simulink model "xo_test"  (R2023a)
settings: Solver=VariableStepAuto  StartTime=0.0  StopTime=10.0  RelTol=1e-3
PreLoadFcn:
  | xo = importrobot('urdf/alpha4_LC_FB_XYZ.urdf');
  | xo.DataFormat = 'col';
libraries: robotmaniplib x72, RoboticsCode x72
(part 1 of 2)
settings Model: Creator=kgross  LastModifiedBy=kgross

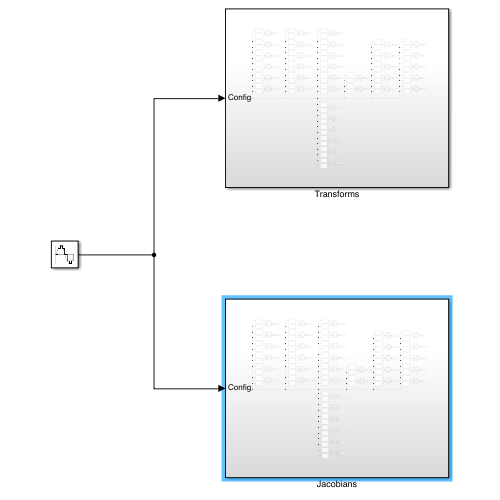
[thumbnail: Simulink's stored preview of the top-level diagram]
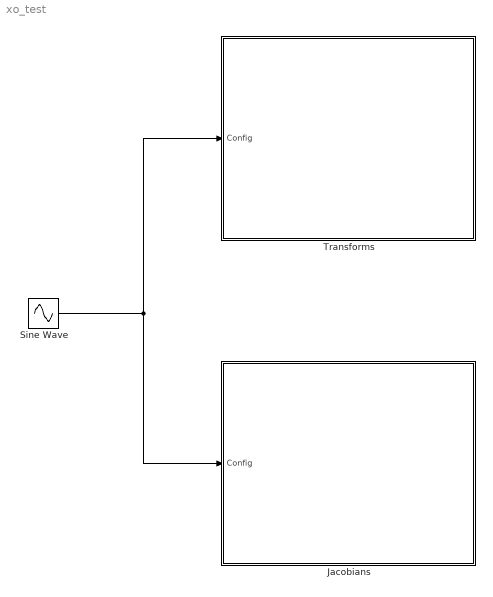
== system xo_test ==
  Jacobians : Subsystem
  Sine Wave : Sin  Amplitude=1:30  Frequency=1:30  SampleTime=0.001
  Transforms : Subsystem
  wires:
  Sine Wave/1 -> Transforms/1(Config), Jacobians/1(Config)

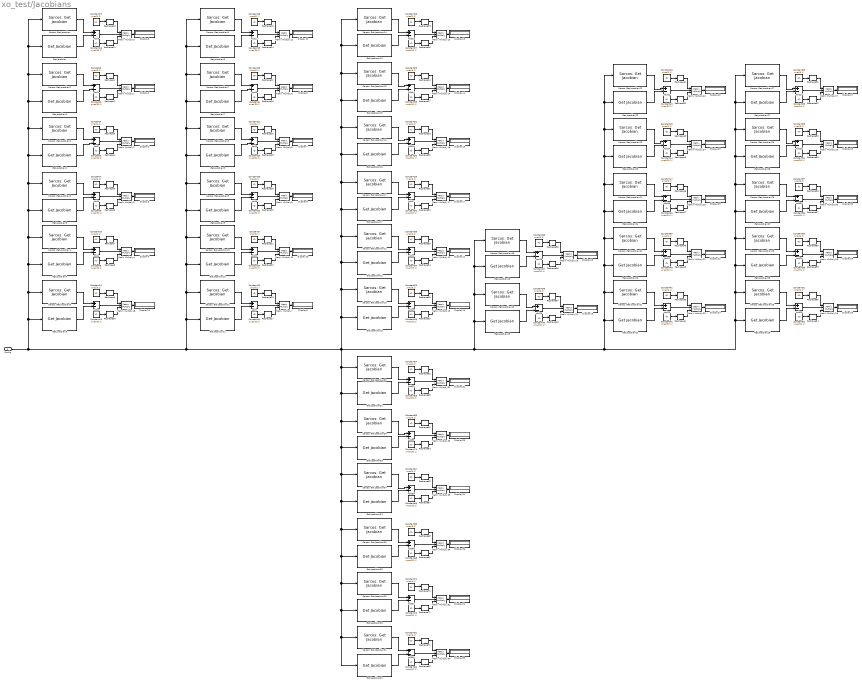
== system xo_test/Jacobians ==
  Config : Inport
  Add{1..36} (36 alike) : Sum  Inputs=+-
  Constant{1,3,5..6,8,13..16,20,22,24,26..27,30,32,34..35,37,40,42,44,46,48..49,52,54,56,58..59,62..63,66,68,70..71} (36 alike) : Constant  Value=ones(30,1)
  Constant{2,4,7,9..12,17..19,21,23,25,28..29,31,33,36,38..39,41,43,45,47,50..51,53,55,57,60..61,64..65,67,69,72} (36 alike) : Constant  Value=ones(6,1)
  Display{1..36} (36 alike) : Display
  Get Jacobian : robotmaniplib/Get Jacobian  RigidBodyTree=xo  EndEffector=BasePosX  SimulateUsing=Interpreted execution
  Get Jacobian1 : robotmaniplib/Get Jacobian  RigidBodyTree=xo  EndEffector=BasePosY  SimulateUsing=Interpreted execution
  Get Jacobian10 : robotmaniplib/Get Jacobian  RigidBodyTree=xo  EndEffector=LeftCalfRotate  SimulateUsing=Interpreted execution
  Get Jacobian11 : robotmaniplib/Get Jacobian  RigidBodyTree=xo  EndEffector=LeftAnkleFlex  SimulateUsing=Interpreted execution
  Get Jacobian12 : robotmaniplib/Get Jacobian  RigidBodyTree=xo  EndEffector=RightCalfRotate  SimulateUsing=Interpreted execution
  Get Jacobian13 : robotmaniplib/Get Jacobian  RigidBodyTree=xo  EndEffector=RightAnkleFlex  SimulateUsing=Interpreted execution
  Get Jacobian14 : robotmaniplib/Get Jacobian  RigidBodyTree=xo  EndEffector=RightHipRotate  SimulateUsing=Interpreted execution
  Get Jacobian15 : robotmaniplib/Get Jacobian  RigidBodyTree=xo  EndEffector=RightHipAbAd  SimulateUsing=Interpreted execution
  Get Jacobian16 : robotmaniplib/Get Jacobian  RigidBodyTree=xo  EndEffector=RightHipFlex  SimulateUsing=Interpreted execution
  Get Jacobian17 : robotmaniplib/Get Jacobian  RigidBodyTree=xo  EndEffector=RightKneeFlex  SimulateUsing=Interpreted execution
  Get Jacobian18 : robotmaniplib/Get Jacobian  RigidBodyTree=xo  EndEffector=TorsoTilt  SimulateUsing=Interpreted execution
  Get Jacobian19 : robotmaniplib/Get Jacobian  RigidBodyTree=xo  EndEffector=TorsoRotate  SimulateUsing=Interpreted execution
  Get Jacobian2 : robotmaniplib/Get Jacobian  RigidBodyTree=xo  EndEffector=BasePosZ  SimulateUsing=Interpreted execution
  Get Jacobian20 : robotmaniplib/Get Jacobian  RigidBodyTree=xo  EndEffector=LeftElbowFlex  SimulateUsing=Interpreted execution
  Get Jacobian21 : robotmaniplib/Get Jacobian  RigidBodyTree=xo  EndEffector=LeftWristRotate  SimulateUsing=Interpreted execution
  Get Jacobian22 : robotmaniplib/Get Jacobian  RigidBodyTree=xo  EndEffector=LeftShoulderAbAd  SimulateUsing=Interpreted execution
  Get Jacobian23 : robotmaniplib/Get Jacobian  RigidBodyTree=xo  EndEffector=LeftShoulderFlex  SimulateUsing=Interpreted execution
  Get Jacobian24 : robotmaniplib/Get Jacobian  RigidBodyTree=xo  EndEffector=LeftHumeralRotate  SimulateUsing=Interpreted execution
  Get Jacobian25 : robotmaniplib/Get Jacobian  RigidBodyTree=xo  EndEffector=RightElbowFlex  SimulateUsing=Interpreted execution
  Get Jacobian26 : robotmaniplib/Get Jacobian  RigidBodyTree=xo  EndEffector=RightWristRotate  SimulateUsing=Interpreted execution
  Get Jacobian27 : robotmaniplib/Get Jacobian  RigidBodyTree=xo  EndEffector=RightShoulderAbAd  SimulateUsing=Interpreted execution
  Get Jacobian28 : robotmaniplib/Get Jacobian  RigidBodyTree=xo  EndEffector=RightShoulderFlex  SimulateUsing=Interpreted execution
  Get Jacobian29 : robotmaniplib/Get Jacobian  RigidBodyTree=xo  EndEffector=RightHumeralRotate  SimulateUsing=Interpreted execution
  Get Jacobian3 : robotmaniplib/Get Jacobian  RigidBodyTree=xo  EndEffector=BaseRotX  SimulateUsing=Interpreted execution
  Get Jacobian30 : robotmaniplib/Get Jacobian  RigidBodyTree=xo  EndEffector=LeftHandleLoadCell  SimulateUsing=Interpreted execution
  Get Jacobian31 : robotmaniplib/Get Jacobian  RigidBodyTree=xo  EndEffector=RightHandleLoadCell  SimulateUsing=Interpreted execution
  Get Jacobian32 : robotmaniplib/Get Jacobian  RigidBodyTree=xo  EndEffector=PelvisLoadCell  SimulateUsing=Interpreted execution
  Get Jacobian33 : robotmaniplib/Get Jacobian  RigidBodyTree=xo  EndEffector=LeftFootLoadCell  SimulateUsing=Interpreted execution
  Get Jacobian34 : robotmaniplib/Get Jacobian  RigidBodyTree=xo  EndEffector=RightFootLoadCell  SimulateUsing=Interpreted execution
  Get Jacobian35 : robotmaniplib/Get Jacobian  RigidBodyTree=xo  EndEffector=TorsoLoadCell  SimulateUsing=Interpreted execution
  Get Jacobian4 : robotmaniplib/Get Jacobian  RigidBodyTree=xo  EndEffector=BaseRotY  SimulateUsing=Interpreted execution
  Get Jacobian5 : robotmaniplib/Get Jacobian  RigidBodyTree=xo  EndEffector=BaseRotZ  SimulateUsing=Interpreted execution
  Get Jacobian6 : robotmaniplib/Get Jacobian  RigidBodyTree=xo  EndEffector=LeftHipRotate  SimulateUsing=Interpreted execution
  Get Jacobian7 : robotmaniplib/Get Jacobian  RigidBodyTree=xo  EndEffector=LeftHipAbAd  SimulateUsing=Interpreted execution
  Get Jacobian8 : robotmaniplib/Get Jacobian  RigidBodyTree=xo  EndEffector=LeftHipFlex  SimulateUsing=Interpreted execution
  Get Jacobian9 : robotmaniplib/Get Jacobian  RigidBodyTree=xo  EndEffector=LeftKneeFlex  SimulateUsing=Interpreted execution
  Matrix Multiply{1..36} (36 alike) : Product  Inputs=3  Multiplication=Matrix(*)
  Reshape{1,3,5,7,9..10,12..13,16,19,21,23..25,28,31,33,35,37..38,41,43,46,48,50..51,53,56,58,60..62,65,68,70,72} (36 alike) : Reshape  OutputDimensionality=Row vector (2-D)
  Reshape{2,4,6,8,11,14..15,17..18,20,22,26..27,29..30,32,34,36,39..40,42,44..45,47,49,52,54..55,57,59,63..64,66..67,69,71} (36 alike) : Reshape  OutputDimensionality=Column vector (2-D)
  Sarcos: Get Jacobian : RoboticsCode/Sarcos: Get Jacobian  urdfpath='alpha4_LC_FB_XYZ.urdf'  source=BasePosX  source_string='BasePosX'  names_length=30
      settings: SourceProductName=Sacros Robotics Toolbox
  Sarcos: Get Jacobian1 : RoboticsCode/Sarcos: Get Jacobian  urdfpath='alpha4_LC_FB_XYZ.urdf'  source=BasePosY  source_string='BasePosY'  names_length=30
      settings: SourceProductName=Sacros Robotics Toolbox
  Sarcos: Get Jacobian10 : RoboticsCode/Sarcos: Get Jacobian  urdfpath='alpha4_LC_FB_XYZ.urdf'  source=LeftCalfRotate  source_string='LeftCalfRotate'  names_length=30
      settings: SourceProductName=Sacros Robotics Toolbox
  Sarcos: Get Jacobian11 : RoboticsCode/Sarcos: Get Jacobian  urdfpath='alpha4_LC_FB_XYZ.urdf'  source=LeftAnkleFlex  source_string='LeftAnkleFlex'  names_length=30
      settings: SourceProductName=Sacros Robotics Toolbox
  Sarcos: Get Jacobian12 : RoboticsCode/Sarcos: Get Jacobian  urdfpath='alpha4_LC_FB_XYZ.urdf'  source=RightCalfRotate  source_string='RightCalfRotate'  names_length=30
      settings: SourceProductName=Sacros Robotics Toolbox
  Sarcos: Get Jacobian13 : RoboticsCode/Sarcos: Get Jacobian  urdfpath='alpha4_LC_FB_XYZ.urdf'  source=RightAnkleFlex  source_string='RightAnkleFlex'  names_length=30
      settings: SourceProductName=Sacros Robotics Toolbox
  Sarcos: Get Jacobian14 : RoboticsCode/Sarcos: Get Jacobian  urdfpath='alpha4_LC_FB_XYZ.urdf'  source=RightHipRotate  source_string='RightHipRotate'  names_length=30
      settings: SourceProductName=Sacros Robotics Toolbox
  Sarcos: Get Jacobian15 : RoboticsCode/Sarcos: Get Jacobian  urdfpath='alpha4_LC_FB_XYZ.urdf'  source=RightHipAbAd  source_string='RightHipAbAd'  names_length=30
      settings: SourceProductName=Sacros Robotics Toolbox
  Sarcos: Get Jacobian16 : RoboticsCode/Sarcos: Get Jacobian  urdfpath='alpha4_LC_FB_XYZ.urdf'  source=RightHipFlex  source_string='RightHipFlex'  names_length=30
      settings: SourceProductName=Sacros Robotics Toolbox
  Sarcos: Get Jacobian17 : RoboticsCode/Sarcos: Get Jacobian  urdfpath='alpha4_LC_FB_XYZ.urdf'  source=RightKneeFlex  source_string='RightKneeFlex'  names_length=30
      settings: SourceProductName=Sacros Robotics Toolbox
  Sarcos: Get Jacobian18 : RoboticsCode/Sarcos: Get Jacobian  urdfpath='alpha4_LC_FB_XYZ.urdf'  source=TorsoTilt  source_string='TorsoTilt'  names_length=30
      settings: SourceProductName=Sacros Robotics Toolbox
  Sarcos: Get Jacobian19 : RoboticsCode/Sarcos: Get Jacobian  urdfpath='alpha4_LC_FB_XYZ.urdf'  source=TorsoRotate  source_string='TorsoRotate'  names_length=30
      settings: SourceProductName=Sacros Robotics Toolbox
  Sarcos: Get Jacobian2 : RoboticsCode/Sarcos: Get Jacobian  urdfpath='alpha4_LC_FB_XYZ.urdf'  source=BasePosZ  source_string='BasePosZ'  names_length=30
      settings: SourceProductName=Sacros Robotics Toolbox
  Sarcos: Get Jacobian20 : RoboticsCode/Sarcos: Get Jacobian  urdfpath='alpha4_LC_FB_XYZ.urdf'  source=LeftElbowFlex  source_string='LeftElbowFlex'  names_length=30
      settings: SourceProductName=Sacros Robotics Toolbox
  Sarcos: Get Jacobian21 : RoboticsCode/Sarcos: Get Jacobian  urdfpath='alpha4_LC_FB_XYZ.urdf'  source=LeftWristRotate  source_string='LeftWristRotate'  names_length=30
      settings: SourceProductName=Sacros Robotics Toolbox
  Sarcos: Get Jacobian22 : RoboticsCode/Sarcos: Get Jacobian  urdfpath='alpha4_LC_FB_XYZ.urdf'  source=LeftShoulderAbAd  source_string='LeftShoulderAbAd'  names_length=30
      settings: SourceProductName=Sacros Robotics Toolbox
  Sarcos: Get Jacobian23 : RoboticsCode/Sarcos: Get Jacobian  urdfpath='alpha4_LC_FB_XYZ.urdf'  source=LeftShoulderFlex  source_string='LeftShoulderFlex'  names_length=30
      settings: SourceProductName=Sacros Robotics Toolbox
  Sarcos: Get Jacobian24 : RoboticsCode/Sarcos: Get Jacobian  urdfpath='alpha4_LC_FB_XYZ.urdf'  source=LeftHumeralRotate  source_string='LeftHumeralRotate'  names_length=30
      settings: SourceProductName=Sacros Robotics Toolbox
  Sarcos: Get Jacobian25 : RoboticsCode/Sarcos: Get Jacobian  urdfpath='alpha4_LC_FB_XYZ.urdf'  source=RightElbowFlex  source_string='RightElbowFlex'  names_length=30
      settings: SourceProductName=Sacros Robotics Toolbox
  Sarcos: Get Jacobian26 : RoboticsCode/Sarcos: Get Jacobian  urdfpath='alpha4_LC_FB_XYZ.urdf'  source=RightWristRotate  source_string='RightWristRotate'  names_length=30
      settings: SourceProductName=Sacros Robotics Toolbox
  Sarcos: Get Jacobian27 : RoboticsCode/Sarcos: Get Jacobian  urdfpath='alpha4_LC_FB_XYZ.urdf'  source=RightShoulderAbAd  source_string='RightShoulderAbAd'  names_length=30
      settings: SourceProductName=Sacros Robotics Toolbox
  Sarcos: Get Jacobian28 : RoboticsCode/Sarcos: Get Jacobian  urdfpath='alpha4_LC_FB_XYZ.urdf'  source=RightShoulderFlex  source_string='RightShoulderFlex'  names_length=30
      settings: SourceProductName=Sacros Robotics Toolbox
  Sarcos: Get Jacobian29 : RoboticsCode/Sarcos: Get Jacobian  urdfpath='alpha4_LC_FB_XYZ.urdf'  source=RightHumeralRotate  source_string='RightHumeralRotate'  names_length=30
      settings: SourceProductName=Sacros Robotics Toolbox
  Sarcos: Get Jacobian3 : RoboticsCode/Sarcos: Get Jacobian  urdfpath='alpha4_LC_FB_XYZ.urdf'  source=BaseRotX  source_string='BaseRotX'  names_length=30
      settings: SourceProductName=Sacros Robotics Toolbox
  Sarcos: Get Jacobian30 : RoboticsCode/Sarcos: Get Jacobian  urdfpath='alpha4_LC_FB_XYZ.urdf'  source=LeftHandleLoadCell  source_string='LeftHandleLoadCell'  names_length=30
      settings: SourceProductName=Sacros Robotics Toolbox
  Sarcos: Get Jacobian31 : RoboticsCode/Sarcos: Get Jacobian  urdfpath='alpha4_LC_FB_XYZ.urdf'  source=RightHandleLoadCell  source_string='RightHandleLoadCell'  names_length=30
      settings: SourceProductName=Sacros Robotics Toolbox
  Sarcos: Get Jacobian32 : RoboticsCode/Sarcos: Get Jacobian  urdfpath='alpha4_LC_FB_XYZ.urdf'  source=PelvisLoadCell  source_string='PelvisLoadCell'  names_length=30
      settings: SourceProductName=Sacros Robotics Toolbox
  Sarcos: Get Jacobian33 : RoboticsCode/Sarcos: Get Jacobian  urdfpath='alpha4_LC_FB_XYZ.urdf'  source=LeftFootLoadCell  source_string='LeftFootLoadCell'  names_length=30
      settings: SourceProductName=Sacros Robotics Toolbox
  Sarcos: Get Jacobian34 : RoboticsCode/Sarcos: Get Jacobian  urdfpath='alpha4_LC_FB_XYZ.urdf'  source=RightFootLoadCell  source_string='RightFootLoadCell'  names_length=30
      settings: SourceProductName=Sacros Robotics Toolbox
  Sarcos: Get Jacobian35 : RoboticsCode/Sarcos: Get Jacobian  urdfpath='alpha4_LC_FB_XYZ.urdf'  source=TorsoLoadCell  source_string='TorsoLoadCell'  names_length=30
      settings: SourceProductName=Sacros Robotics Toolbox
  Sarcos: Get Jacobian4 : RoboticsCode/Sarcos: Get Jacobian  urdfpath='alpha4_LC_FB_XYZ.urdf'  source=BaseRotY  source_string='BaseRotY'  names_length=30
      settings: SourceProductName=Sacros Robotics Toolbox
  Sarcos: Get Jacobian5 : RoboticsCode/Sarcos: Get Jacobian  urdfpath='alpha4_LC_FB_XYZ.urdf'  source=BaseRotZ  source_string='BaseRotZ'  names_length=30
      settings: SourceProductName=Sacros Robotics Toolbox
  Sarcos: Get Jacobian6 : RoboticsCode/Sarcos: Get Jacobian  urdfpath='alpha4_LC_FB_XYZ.urdf'  source=LeftHipRotate  source_string='LeftHipRotate'  names_length=30
      settings: SourceProductName=Sacros Robotics Toolbox
  Sarcos: Get Jacobian7 : RoboticsCode/Sarcos: Get Jacobian  urdfpath='alpha4_LC_FB_XYZ.urdf'  source=LeftHipAbAd  source_string='LeftHipAbAd'  names_length=30
      settings: SourceProductName=Sacros Robotics Toolbox
  Sarcos: Get Jacobian8 : RoboticsCode/Sarcos: Get Jacobian  urdfpath='alpha4_LC_FB_XYZ.urdf'  source=LeftHipFlex  source_string='LeftHipFlex'  names_length=30
      settings: SourceProductName=Sacros Robotics Toolbox
  Sarcos: Get Jacobian9 : RoboticsCode/Sarcos: Get Jacobian  urdfpath='alpha4_LC_FB_XYZ.urdf'  source=LeftKneeFlex  source_string='LeftKneeFlex'  names_length=30
      settings: SourceProductName=Sacros Robotics Toolbox
  wires:
  Get Jacobian3/1 -> Add3/2
  Sarcos: Get Jacobian4/1 -> Add4/1
  Get Jacobian4/1 -> Add4/2
  Get Jacobian2/1 -> Add2/2
  Sarcos: Get Jacobian1/1 -> Add1/1
  Get Jacobian1/1 -> Add1/2
  Add5/1 -> Matrix Multiply5/2
  Sarcos: Get Jacobian/1 -> Add5/1
  Get Jacobian/1 -> Add5/2
  Reshape11/1 -> Matrix Multiply5/3
  Get Jacobian5/1 -> Add18/2
  Sarcos: Get Jacobian9/1 -> Add9/1
  Get Jacobian9/1 -> Add9/2
  Sarcos: Get Jacobian10/1 -> Add10/1
  Sarcos: Get Jacobian2/1 -> Add2/1
  Get Jacobian6/1 -> Add11/2
  Get Jacobian8/1 -> Add8/2
  Sarcos: Get Jacobian8/1 -> Add8/1
  Get Jacobian11/1 -> Add7/2
  Sarcos: Get Jacobian11/1 -> Add7/1
  Matrix Multiply5/1 -> Display5/1
  Get Jacobian10/1 -> Add10/2
  Sarcos: Get Jacobian14/1 -> Add13/1
  Get Jacobian15/1 -> Add14/2
  Get Jacobian12/1 -> Add12/2
  Constant16/1 -> Reshape11/1
  Constant17/1 -> Reshape10/1
  Sarcos: Get Jacobian12/1 -> Add12/1
  Sarcos: Get Jacobian15/1 -> Add14/1
  Get Jacobian17/1 -> Add17/2
  Sarcos: Get Jacobian5/1 -> Add18/1
  Sarcos: Get Jacobian17/1 -> Add17/1
  Get Jacobian13/1 -> Add15/2
  Sarcos: Get Jacobian3/1 -> Add3/1
  Get Jacobian16/1 -> Add16/2
  Sarcos: Get Jacobian6/1 -> Add11/1
  Sarcos: Get Jacobian13/1 -> Add15/1
  Sarcos: Get Jacobian7/1 -> Add6/1
  Get Jacobian7/1 -> Add6/2
  Get Jacobian14/1 -> Add13/2
  Reshape10/1 -> Matrix Multiply5/1
  Sarcos: Get Jacobian16/1 -> Add16/1
  Reshape1/1 -> Matrix Multiply1/1
  Constant2/1 -> Reshape1/1
  Constant1/1 -> Reshape2/1
  Matrix Multiply1/1 -> Display1/1
  Reshape2/1 -> Matrix Multiply1/3
  Add1/1 -> Matrix Multiply1/2
  Add2/1 -> Matrix Multiply2/2
  Reshape4/1 -> Matrix Multiply2/3
  Matrix Multiply2/1 -> Display2/1
  Constant3/1 -> Reshape4/1
  Constant4/1 -> Reshape3/1
  Reshape3/1 -> Matrix Multiply2/1
  Reshape5/1 -> Matrix Multiply3/1
  Constant7/1 -> Reshape5/1
  Constant5/1 -> Reshape6/1
  Matrix Multiply3/1 -> Display3/1
  Reshape6/1 -> Matrix Multiply3/3
  Add3/1 -> Matrix Multiply3/2
  Add4/1 -> Matrix Multiply4/2
  Reshape8/1 -> Matrix Multiply4/3
  Matrix Multiply4/1 -> Display4/1
  Constant8/1 -> Reshape8/1
  Constant10/1 -> Reshape7/1
  Reshape7/1 -> Matrix Multiply4/1
  Reshape9/1 -> Matrix Multiply18/1
  Constant11/1 -> Reshape9/1
  Constant13/1 -> Reshape36/1
  Matrix Multiply18/1 -> Display20/1
  Reshape36/1 -> Matrix Multiply18/3
  Add18/1 -> Matrix Multiply18/2
  Add7/1 -> Matrix Multiply7/2
  Reshape17/1 -> Matrix Multiply7/3
  Matrix Multiply7/1 -> Display8/1
  Constant14/1 -> Reshape17/1
  Constant12/1 -> Reshape23/1
  Reshape23/1 -> Matrix Multiply7/1
  Reshape21/1 -> Matrix Multiply10/1
  Constant9/1 -> Reshape21/1
  Constant24/1 -> Reshape22/1
  Matrix Multiply10/1 -> Display10/1
  Reshape22/1 -> Matrix Multiply10/3
  Add10/1 -> Matrix Multiply10/2
  Add9/1 -> Matrix Multiply9/2
  Reshape20/1 -> Matrix Multiply9/3
  Matrix Multiply9/1 -> Display9/1
  Constant22/1 -> Reshape20/1
  Constant23/1 -> Reshape19/1
  Reshape19/1 -> Matrix Multiply9/1
  Reshape16/1 -> Matrix Multiply8/1
  Constant21/1 -> Reshape16/1
  Constant20/1 -> Reshape18/1
  Matrix Multiply8/1 -> Display7/1
  Reshape18/1 -> Matrix Multiply8/3
  Add8/1 -> Matrix Multiply8/2
  Add6/1 -> Matrix Multiply6/2
  Reshape15/1 -> Matrix Multiply6/3
  Matrix Multiply6/1 -> Display6/1
  Constant6/1 -> Reshape15/1
  Constant19/1 -> Reshape12/1
  Reshape12/1 -> Matrix Multiply6/1
  Reshape13/1 -> Matrix Multiply11/1
  Constant18/1 -> Reshape13/1
  Constant15/1 -> Reshape14/1
  Matrix Multiply11/1 -> Display11/1
  Reshape14/1 -> Matrix Multiply11/3
  Add11/1 -> Matrix Multiply11/2
  Add13/1 -> Matrix Multiply13/2
  Reshape26/1 -> Matrix Multiply13/3
  Matrix Multiply13/1 -> Display13/1
  Constant27/1 -> Reshape26/1
  Constant28/1 -> Reshape25/1
  Reshape25/1 -> Matrix Multiply13/1
  Reshape24/1 -> Matrix Multiply14/1
  Constant29/1 -> Reshape24/1
  Constant35/1 -> Reshape27/1
  Matrix Multiply14/1 -> Display14/1
  Reshape27/1 -> Matrix Multiply14/3
  Add14/1 -> Matrix Multiply14/2
  Add16/1 -> Matrix Multiply16/2
  Reshape30/1 -> Matrix Multiply16/3
  Matrix Multiply16/1 -> Display15/1
  Constant30/1 -> Reshape30/1
  Constant31/1 -> Reshape28/1
  Reshape28/1 -> Matrix Multiply16/1
  Reshape31/1 -> Matrix Multiply17/1
  Constant33/1 -> Reshape31/1
  Constant32/1 -> Reshape32/1
  Matrix Multiply17/1 -> Display17/1
  Reshape32/1 -> Matrix Multiply17/3
  Add17/1 -> Matrix Multiply17/2
  Add12/1 -> Matrix Multiply12/2
  Reshape34/1 -> Matrix Multiply12/3
  Matrix Multiply12/1 -> Display12/1
  Constant34/1 -> Reshape34/1
  Constant36/1 -> Reshape33/1
  Reshape33/1 -> Matrix Multiply12/1
  Reshape35/1 -> Matrix Multiply15/1
  Constant25/1 -> Reshape35/1
  Constant26/1 -> Reshape29/1
  Matrix Multiply15/1 -> Display16/1
  Reshape29/1 -> Matrix Multiply15/3
  Add15/1 -> Matrix Multiply15/2
  Add20/1 -> Matrix Multiply20/2
  Reshape40/1 -> Matrix Multiply20/3
  Matrix Multiply20/1 -> Display19/1
  Constant40/1 -> Reshape40/1
  Constant39/1 -> Reshape37/1
  Reshape37/1 -> Matrix Multiply20/1
  Reshape38/1 -> Matrix Multiply19/1
  Constant38/1 -> Reshape38/1
  Constant37/1 -> Reshape39/1
  Matrix Multiply19/1 -> Display18/1
  Reshape39/1 -> Matrix Multiply19/3
  Add19/1 -> Matrix Multiply19/2
  Get Jacobian18/1 -> Add19/2
  Sarcos: Get Jacobian19/1 -> Add20/1
  Get Jacobian19/1 -> Add20/2
  Sarcos: Get Jacobian18/1 -> Add19/1
  Add23/1 -> Matrix Multiply23/2
  Reshape44/1 -> Matrix Multiply23/3
  Matrix Multiply23/1 -> Display24/1
  Constant42/1 -> Reshape44/1
  Constant41/1 -> Reshape50/1
  Reshape50/1 -> Matrix Multiply23/1
  Reshape48/1 -> Matrix Multiply21/1
  Constant50/1 -> Reshape48/1
  Constant48/1 -> Reshape49/1
  Matrix Multiply21/1 -> Display21/1
  Reshape49/1 -> Matrix Multiply21/3
  Add21/1 -> Matrix Multiply21/2
  Add25/1 -> Matrix Multiply25/2
  Reshape47/1 -> Matrix Multiply25/3
  Matrix Multiply25/1 -> Display25/1
  Constant46/1 -> Reshape47/1
  Constant47/1 -> Reshape46/1
  Reshape46/1 -> Matrix Multiply25/1
  Reshape43/1 -> Matrix Multiply24/1
  Constant45/1 -> Reshape43/1
  Constant44/1 -> Reshape45/1
  Matrix Multiply24/1 -> Display23/1
  Reshape45/1 -> Matrix Multiply24/3
  Add24/1 -> Matrix Multiply24/2
  Add22/1 -> Matrix Multiply22/2
  Reshape42/1 -> Matrix Multiply22/3
  Matrix Multiply22/1 -> Display22/1
  Constant49/1 -> Reshape42/1
  Constant43/1 -> Reshape41/1
  Reshape41/1 -> Matrix Multiply22/1
  Sarcos: Get Jacobian23/1 -> Add24/1
  Sarcos: Get Jacobian21/1 -> Add23/1
  Get Jacobian23/1 -> Add24/2
  Get Jacobian21/1 -> Add23/2
  Sarcos: Get Jacobian24/1 -> Add25/1
  Get Jacobian24/1 -> Add25/2
  Sarcos: Get Jacobian22/1 -> Add22/1
  Sarcos: Get Jacobian20/1 -> Add21/1
  Get Jacobian20/1 -> Add21/2
  Get Jacobian22/1 -> Add22/2
  Get Jacobian27/1 -> Add27/2
  Get Jacobian25/1 -> Add26/2
  Sarcos: Get Jacobian25/1 -> Add26/1
  Sarcos: Get Jacobian27/1 -> Add27/1
  Get Jacobian29/1 -> Add30/2
  Sarcos: Get Jacobian29/1 -> Add30/1
  Get Jacobian26/1 -> Add28/2
  Get Jacobian28/1 -> Add29/2
  Sarcos: Get Jacobian26/1 -> Add28/1
  Sarcos: Get Jacobian28/1 -> Add29/1
  Reshape51/1 -> Matrix Multiply27/1
  Constant53/1 -> Reshape51/1
  Constant59/1 -> Reshape52/1
  Matrix Multiply27/1 -> Display27/1
  Reshape52/1 -> Matrix Multiply27/3
  Add27/1 -> Matrix Multiply27/2
  Add29/1 -> Matrix Multiply29/2
  Reshape55/1 -> Matrix Multiply29/3
  Matrix Multiply29/1 -> Display28/1
  Constant54/1 -> Reshape55/1
  Constant55/1 -> Reshape53/1
  Reshape53/1 -> Matrix Multiply29/1
  Reshape56/1 -> Matrix Multiply30/1
  Constant57/1 -> Reshape56/1
  Constant56/1 -> Reshape57/1
  Matrix Multiply30/1 -> Display30/1
  Reshape57/1 -> Matrix Multiply30/3
  Add30/1 -> Matrix Multiply30/2
  Add26/1 -> Matrix Multiply26/2
  Reshape59/1 -> Matrix Multiply26/3
  Matrix Multiply26/1 -> Display26/1
  Constant58/1 -> Reshape59/1
  Constant60/1 -> Reshape58/1
  Reshape58/1 -> Matrix Multiply26/1
  Reshape60/1 -> Matrix Multiply28/1
  Constant51/1 -> Reshape60/1
  Constant52/1 -> Reshape54/1
  Matrix Multiply28/1 -> Display29/1
  Reshape54/1 -> Matrix Multiply28/3
  Add28/1 -> Matrix Multiply28/2
  Config/1 -> Get Jacobian10/1, Sarcos: Get Jacobian10/1, Get Jacobian8/1, Sarcos: Get Jacobian8/1, Get Jacobian7/1, Sarcos: Get Jacobian7/1, Sarcos: Get Jacobian6/1, Get Jacobian6/1, Sarcos: Get Jacobian9/1, Get Jacobian9/1, Sarcos: Get Jacobian11/1, Get Jacobian11/1, Get Jacobian31/1, Sarcos: Get Jacobian31/1, Get Jacobian30/1, Sarcos: Get Jacobian30/1, Get Jacobian35/1, Sarcos: Get Jacobian35/1, Get Jacobian34/1, Sarcos: Get Jacobian34/1, Get Jacobian33/1, Sarcos: Get Jacobian33/1, Get Jacobian32/1, Sarcos: Get Jacobian32/1, Sarcos: Get Jacobian27/1, Get Jacobian27/1, Sarcos: Get Jacobian28/1, Get Jacobian28/1, Sarcos: Get Jacobian29/1, Get Jacobian29/1, Sarcos: Get Jacobian25/1, Get Jacobian25/1, Sarcos: Get Jacobian26/1, Get Jacobian26/1, Sarcos: Get Jacobian22/1, Get Jacobian22/1, Sarcos: Get Jacobian23/1, Get Jacobian23/1, Sarcos: Get Jacobian24/1, Get Jacobian24/1, Sarcos: Get Jacobian20/1, Get Jacobian20/1, Sarcos: Get Jacobian21/1, Get Jacobian21/1, Get Jacobian18/1, Sarcos: Get Jacobian18/1, Sarcos: Get Jacobian19/1, Get Jacobian19/1, Get Jacobian12/1, Sarcos: Get Jacobian12/1, Get Jacobian16/1, Sarcos: Get Jacobian16/1, Get Jacobian15/1, Sarcos: Get Jacobian15/1, Sarcos: Get Jacobian14/1, Get Jacobian14/1, Sarcos: Get Jacobian17/1, Get Jacobian17/1, Sarcos: Get Jacobian13/1, Get Jacobian13/1, Get Jacobian4/1, Sarcos: Get Jacobian4/1, Sarcos: Get Jacobian/1, Get Jacobian/1, Sarcos: Get Jacobian1/1, Get Jacobian1/1, Sarcos: Get Jacobian2/1, Get Jacobian2/1, Sarcos: Get Jacobian3/1, Get Jacobian3/1, Sarcos: Get Jacobian5/1, Get Jacobian5/1
  Add34/1 -> Matrix Multiply34/2
  Reshape66/1 -> Matrix Multiply34/3
  Matrix Multiply34/1 -> Display35/1
  Constant62/1 -> Reshape66/1
  Constant61/1 -> Reshape72/1
  Reshape72/1 -> Matrix Multiply34/1
  Reshape70/1 -> Matrix Multiply31/1
  Constant72/1 -> Reshape70/1
  Constant70/1 -> Reshape71/1
  Matrix Multiply31/1 -> Display31/1
  Reshape71/1 -> Matrix Multiply31/3
  Add31/1 -> Matrix Multiply31/2
  Add36/1 -> Matrix Multiply36/2
  Reshape69/1 -> Matrix Multiply36/3
  Matrix Multiply36/1 -> Display36/1
  Constant68/1 -> Reshape69/1
  Constant69/1 -> Reshape68/1
  Reshape68/1 -> Matrix Multiply36/1
  Reshape65/1 -> Matrix Multiply35/1
  Constant67/1 -> Reshape65/1
  Constant66/1 -> Reshape67/1
  Matrix Multiply35/1 -> Display34/1
  Reshape67/1 -> Matrix Multiply35/3
  Add35/1 -> Matrix Multiply35/2
  Add33/1 -> Matrix Multiply33/2
  Reshape64/1 -> Matrix Multiply33/3
  Matrix Multiply33/1 -> Display33/1
  Constant71/1 -> Reshape64/1
  Constant65/1 -> Reshape61/1
  Reshape61/1 -> Matrix Multiply33/1
  Reshape62/1 -> Matrix Multiply32/1
  Constant64/1 -> Reshape62/1
  Constant63/1 -> Reshape63/1
  Matrix Multiply32/1 -> Display32/1
  Reshape63/1 -> Matrix Multiply32/3
  Add32/1 -> Matrix Multiply32/2
  Sarcos: Get Jacobian34/1 -> Add35/1
  Get Jacobian32/1 -> Add32/2
  Sarcos: Get Jacobian31/1 -> Add34/1
  Get Jacobian34/1 -> Add35/2
  Get Jacobian31/1 -> Add34/2
  Sarcos: Get Jacobian35/1 -> Add36/1
  Get Jacobian35/1 -> Add36/2
  Sarcos: Get Jacobian33/1 -> Add33/1
  Sarcos: Get Jacobian30/1 -> Add31/1
  Get Jacobian30/1 -> Add31/2
  Get Jacobian33/1 -> Add33/2
  Sarcos: Get Jacobian32/1 -> Add32/1
